simulink model "clusterDemo"  (Simulink 7.4)
settings: Solver=ode45  StartTime=0.0  StopTime=10.0  RelTol=1e-3
values from neighbouring files (symbols this model uses):
  A = 1    [clusterDemo.mat]
  B = [-1 -1 -1 -1 -1 -1 -1 -1 -1 -1 -1 -1 ... (21 elements, 1x21)]    [clusterDemo.mat]
  C = 1    [clusterDemo.mat]
  D = [0 0 0 0 0 0 0 0 0 0 0 0 ... (21 elements, 1x21)]    [clusterDemo.mat]
  N = 5    [clusterDemo.mat]    (also in firefliesDemo.mat = 10)
  var = 0    [clusterDemo.mat]    (also in firefliesDemo.mat = 3)
  x0 = 80    [clusterDemo.mat]
(part 1 of 4)
settings Model: Creator=chepeadan  LastModifiedBy=chepeadan
settings DataIOCC: SaveOutput=off  SaveState=on

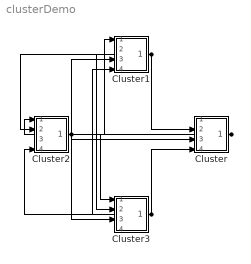
== system clusterDemo ==
  Cluster : Subsystem
  Cluster1 : Subsystem
  Cluster2 : Subsystem
  Cluster3 : Subsystem
  wires:
  Cluster/1(Out1) -> Cluster1/1(In1), Cluster2/1(In1), Cluster3/1(In1)
  Cluster1/1(Out1) -> Cluster/2(In2), Cluster2/2(In2), Cluster3/2(In2)
  Cluster2/1(Out1) -> Cluster/3(In3), Cluster1/3(In3), Cluster3/3(In3)
  Cluster3/1(Out1) -> Cluster/4(In4), Cluster1/4(In4), Cluster2/4(In4)

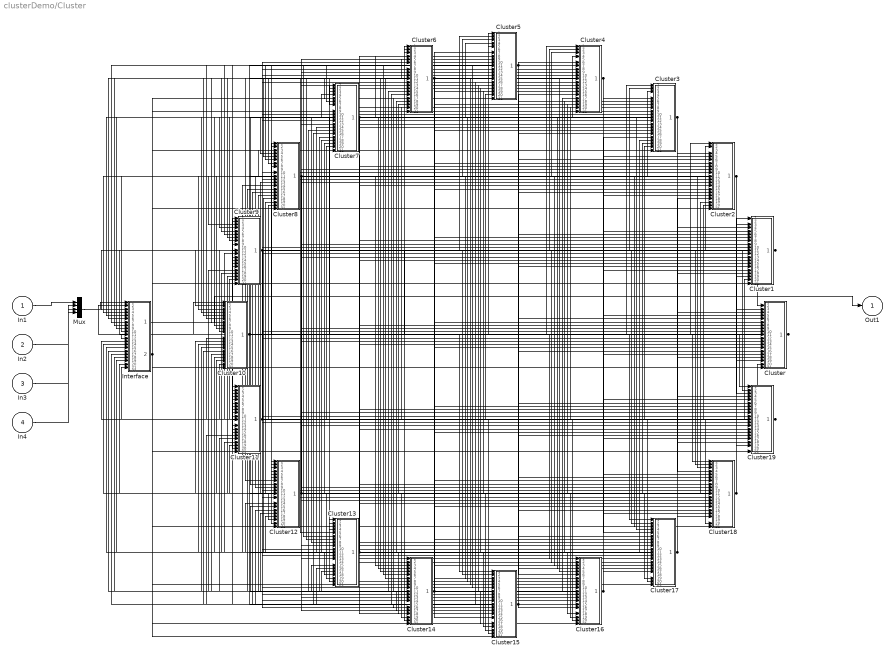
== system clusterDemo/Cluster ==
  In1 : Inport
  In2 : Inport  Port=2
  In3 : Inport  Port=3
  In4 : Inport  Port=4
  Cluster : Subsystem
  Cluster1 : Subsystem
  Cluster10 : Subsystem
  Cluster11 : Subsystem
  Cluster12 : Subsystem
  Cluster13 : Subsystem
  Cluster14 : Subsystem
  Cluster15 : Subsystem
  Cluster16 : Subsystem
  Cluster17 : Subsystem
  Cluster18 : Subsystem
  Cluster19 : Subsystem
  Cluster2 : Subsystem
  Cluster3 : Subsystem
  Cluster4 : Subsystem
  Cluster5 : Subsystem
  Cluster6 : Subsystem
  Cluster7 : Subsystem
  Cluster8 : Subsystem
  Cluster9 : Subsystem
  Interface : Subsystem
  Mux : Mux
  Out1 : Outport
  wires:
  In4/1 -> Mux/4
  In3/1 -> Mux/3
  In2/1 -> Mux/2
  Interface/1(layerOut) -> Out1/1
  Interface/2(Out1) -> Cluster19/21(In21), Cluster18/21(In21), Cluster17/21(In21), Cluster16/21(In21), Cluster15/21(In21), Cluster14/21(In21), Cluster13/21(In21), Cluster12/21(In21), Cluster11/21(In21), Cluster10/21(In21), Cluster9/21(In21), Cluster8/21(In21), Cluster7/21(In21), Cluster6/21(In21), Cluster5/21(In21), Cluster4/21(In21), Cluster3/21(In21), Cluster2/21(In21), Cluster1/21(In21), Cluster/21(In21)
  Cluster19/1(Out1) -> Interface/21(In20), Cluster18/20(In20), Cluster17/20(In20), Cluster16/20(In20), Cluster15/20(In20), Cluster14/20(In20), Cluster13/20(In20), Cluster12/20(In20), Cluster11/20(In20), Cluster10/20(In20), Cluster9/20(In20), Cluster8/20(In20), Cluster7/20(In20), Cluster6/20(In20), Cluster5/20(In20), Cluster4/20(In20), Cluster3/20(In20), Cluster2/20(In20), Cluster1/20(In20), Cluster/20(In20)
  Cluster18/1(Out1) -> Interface/20(In19), Cluster19/19(In19), Cluster17/19(In19), Cluster16/19(In19), Cluster15/19(In19), Cluster14/19(In19), Cluster13/19(In19), Cluster12/19(In19), Cluster11/19(In19), Cluster10/19(In19), Cluster9/19(In19), Cluster8/19(In19), Cluster7/19(In19), Cluster6/19(In19), Cluster5/19(In19), Cluster4/19(In19), Cluster3/19(In19), Cluster2/19(In19), Cluster1/19(In19), Cluster/19(In19)
  Cluster17/1(Out1) -> Interface/19(In18), Cluster19/18(In18), Cluster18/18(In18), Cluster16/18(In18), Cluster15/18(In18), Cluster14/18(In18), Cluster13/18(In18), Cluster12/18(In18), Cluster11/18(In18), Cluster10/18(In18), Cluster9/18(In18), Cluster8/18(In18), Cluster7/18(In18), Cluster6/18(In18), Cluster5/18(In18), Cluster4/18(In18), Cluster3/18(In18), Cluster2/18(In18), Cluster1/18(In18), Cluster/18(In18)
  Cluster16/1(Out1) -> Interface/18(In17), Cluster19/17(In17), Cluster18/17(In17), Cluster17/17(In17), Cluster15/17(In17), Cluster14/17(In17), Cluster13/17(In17), Cluster12/17(In17), Cluster11/17(In17), Cluster10/17(In17), Cluster9/17(In17), Cluster8/17(In17), Cluster7/17(In17), Cluster6/17(In17), Cluster5/17(In17), Cluster4/17(In17), Cluster3/17(In17), Cluster2/17(In17), Cluster1/17(In17), Cluster/17(In17)
  Cluster15/1(Out1) -> Interface/17(In16), Cluster19/16(In16), Cluster18/16(In16), Cluster17/16(In16), Cluster16/16(In16), Cluster14/16(In16), Cluster13/16(In16), Cluster12/16(In16), Cluster11/16(In16), Cluster10/16(In16), Cluster9/16(In16), Cluster8/16(In16), Cluster7/16(In16), Cluster6/16(In16), Cluster5/16(In16), Cluster4/16(In16), Cluster3/16(In16), Cluster2/16(In16), Cluster1/16(In16), Cluster/16(In16)
  Cluster14/1(Out1) -> Interface/16(In15), Cluster19/15(In15), Cluster18/15(In15), Cluster17/15(In15), Cluster16/15(In15), Cluster15/15(In15), Cluster13/15(In15), Cluster12/15(In15), Cluster11/15(In15), Cluster10/15(In15), Cluster9/15(In15), Cluster8/15(In15), Cluster7/15(In15), Cluster6/15(In15), Cluster5/15(In15), Cluster4/15(In15), Cluster3/15(In15), Cluster2/15(In15), Cluster1/15(In15), Cluster/15(In15)
  Cluster13/1(Out1) -> Interface/15(In14), Cluster19/14(In14), Cluster18/14(In14), Cluster17/14(In14), Cluster16/14(In14), Cluster15/14(In14), Cluster14/14(In14), Cluster12/14(In14), Cluster11/14(In14), Cluster10/14(In14), Cluster9/14(In14), Cluster8/14(In14), Cluster7/14(In14), Cluster6/14(In14), Cluster5/14(In14), Cluster4/14(In14), Cluster3/14(In14), Cluster2/14(In14), Cluster1/14(In14), Cluster/14(In14)
  Cluster12/1(Out1) -> Interface/14(In13), Cluster19/13(In13), Cluster18/13(In13), Cluster17/13(In13), Cluster16/13(In13), Cluster15/13(In13), Cluster14/13(In13), Cluster13/13(In13), Cluster11/13(In13), Cluster10/13(In13), Cluster9/13(In13), Cluster8/13(In13), Cluster7/13(In13), Cluster6/13(In13), Cluster5/13(In13), Cluster4/13(In13), Cluster3/13(In13), Cluster2/13(In13), Cluster1/13(In13), Cluster/13(In13)
  Cluster11/1(Out1) -> Interface/13(In12), Cluster19/12(In12), Cluster18/12(In12), Cluster17/12(In12), Cluster16/12(In12), Cluster15/12(In12), Cluster14/12(In12), Cluster13/12(In12), Cluster12/12(In12), Cluster10/12(In12), Cluster9/12(In12), Cluster8/12(In12), Cluster7/12(In12), Cluster6/12(In12), Cluster5/12(In12), Cluster4/12(In12), Cluster3/12(In12), Cluster2/12(In12), Cluster1/12(In12), Cluster/12(In12)
  Cluster10/1(Out1) -> Interface/12(In11), Cluster19/11(In11), Cluster18/11(In11), Cluster17/11(In11), Cluster16/11(In11), Cluster15/11(In11), Cluster14/11(In11), Cluster13/11(In11), Cluster12/11(In11), Cluster11/11(In11), Cluster9/11(In11), Cluster8/11(In11), Cluster7/11(In11), Cluster6/11(In11), Cluster5/11(In11), Cluster4/11(In11), Cluster3/11(In11), Cluster2/11(In11), Cluster1/11(In11), Cluster/11(In11)
  Cluster9/1(Out1) -> Interface/11(In10), Cluster19/10(In10), Cluster18/10(In10), Cluster17/10(In10), Cluster16/10(In10), Cluster15/10(In10), Cluster14/10(In10), Cluster13/10(In10), Cluster12/10(In10), Cluster11/10(In10), Cluster10/10(In10), Cluster8/10(In10), Cluster7/10(In10), Cluster6/10(In10), Cluster5/10(In10), Cluster4/10(In10), Cluster3/10(In10), Cluster2/10(In10), Cluster1/10(In10), Cluster/10(In10)
  Cluster8/1(Out1) -> Interface/10(In9), Cluster19/9(In9), Cluster18/9(In9), Cluster17/9(In9), Cluster16/9(In9), Cluster15/9(In9), Cluster14/9(In9), Cluster13/9(In9), Cluster12/9(In9), Cluster11/9(In9), Cluster10/9(In9), Cluster9/9(In9), Cluster7/9(In9), Cluster6/9(In9), Cluster5/9(In9), Cluster4/9(In9), Cluster3/9(In9), Cluster2/9(In9), Cluster1/9(In9), Cluster/9(In9)
  Cluster7/1(Out1) -> Interface/9(In8), Cluster19/8(In8), Cluster18/8(In8), Cluster17/8(In8), Cluster16/8(In8), Cluster15/8(In8), Cluster14/8(In8), Cluster13/8(In8), Cluster12/8(In8), Cluster11/8(In8), Cluster10/8(In8), Cluster9/8(In8), Cluster8/8(In8), Cluster6/8(In8), Cluster5/8(In8), Cluster4/8(In8), Cluster3/8(In8), Cluster2/8(In8), Cluster1/8(In8), Cluster/8(In8)
  Cluster6/1(Out1) -> Interface/8(In7), Cluster19/7(In7), Cluster18/7(In7), Cluster17/7(In7), Cluster16/7(In7), Cluster15/7(In7), Cluster14/7(In7), Cluster13/7(In7), Cluster12/7(In7), Cluster11/7(In7), Cluster10/7(In7), Cluster9/7(In7), Cluster8/7(In7), Cluster7/7(In7), Cluster5/7(In7), Cluster4/7(In7), Cluster3/7(In7), Cluster2/7(In7), Cluster1/7(In7), Cluster/7(In7)
  Cluster5/1(Out1) -> Interface/7(In6), Cluster19/6(In6), Cluster18/6(In6), Cluster17/6(In6), Cluster16/6(In6), Cluster15/6(In6), Cluster14/6(In6), Cluster13/6(In6), Cluster12/6(In6), Cluster11/6(In6), Cluster10/6(In6), Cluster9/6(In6), Cluster8/6(In6), Cluster7/6(In6), Cluster6/6(In6), Cluster4/6(In6), Cluster3/6(In6), Cluster2/6(In6), Cluster1/6(In6), Cluster/6(In6)
  Cluster4/1(Out1) -> Interface/6(In5), Cluster19/5(In5), Cluster18/5(In5), Cluster17/5(In5), Cluster16/5(In5), Cluster15/5(In5), Cluster14/5(In5), Cluster13/5(In5), Cluster12/5(In5), Cluster11/5(In5), Cluster10/5(In5), Cluster9/5(In5), Cluster8/5(In5), Cluster7/5(In5), Cluster6/5(In5), Cluster5/5(In5), Cluster3/5(In5), Cluster2/5(In5), Cluster1/5(In5), Cluster/5(In5)
  Cluster3/1(Out1) -> Interface/5(In4), Cluster19/4(In4), Cluster18/4(In4), Cluster17/4(In4), Cluster16/4(In4), Cluster15/4(In4), Cluster14/4(In4), Cluster13/4(In4), Cluster12/4(In4), Cluster11/4(In4), Cluster10/4(In4), Cluster9/4(In4), Cluster8/4(In4), Cluster7/4(In4), Cluster6/4(In4), Cluster5/4(In4), Cluster4/4(In4), Cluster2/4(In4), Cluster1/4(In4), Cluster/4(In4)
  Cluster2/1(Out1) -> Interface/4(In3), Cluster19/3(In3), Cluster18/3(In3), Cluster17/3(In3), Cluster16/3(In3), Cluster15/3(In3), Cluster14/3(In3), Cluster13/3(In3), Cluster12/3(In3), Cluster11/3(In3), Cluster10/3(In3), Cluster9/3(In3), Cluster8/3(In3), Cluster7/3(In3), Cluster6/3(In3), Cluster5/3(In3), Cluster4/3(In3), Cluster3/3(In3), Cluster1/3(In3), Cluster/3(In3)
  Cluster1/1(Out1) -> Interface/3(In2), Cluster19/2(In2), Cluster18/2(In2), Cluster17/2(In2), Cluster16/2(In2), Cluster15/2(In2), Cluster14/2(In2), Cluster13/2(In2), Cluster12/2(In2), Cluster11/2(In2), Cluster10/2(In2), Cluster9/2(In2), Cluster8/2(In2), Cluster7/2(In2), Cluster6/2(In2), Cluster5/2(In2), Cluster4/2(In2), Cluster3/2(In2), Cluster2/2(In2), Cluster/2(In2)
  Cluster/1(Out1) -> Interface/2(In1), Cluster19/1(In1), Cluster18/1(In1), Cluster17/1(In1), Cluster16/1(In1), Cluster15/1(In1), Cluster14/1(In1), Cluster13/1(In1), Cluster12/1(In1), Cluster11/1(In1), Cluster10/1(In1), Cluster9/1(In1), Cluster8/1(In1), Cluster7/1(In1), Cluster6/1(In1), Cluster5/1(In1), Cluster4/1(In1), Cluster3/1(In1), Cluster2/1(In1), Cluster1/1(In1)
  In1/1 -> Mux/1
  Mux/1 -> Interface/1(layerIn)

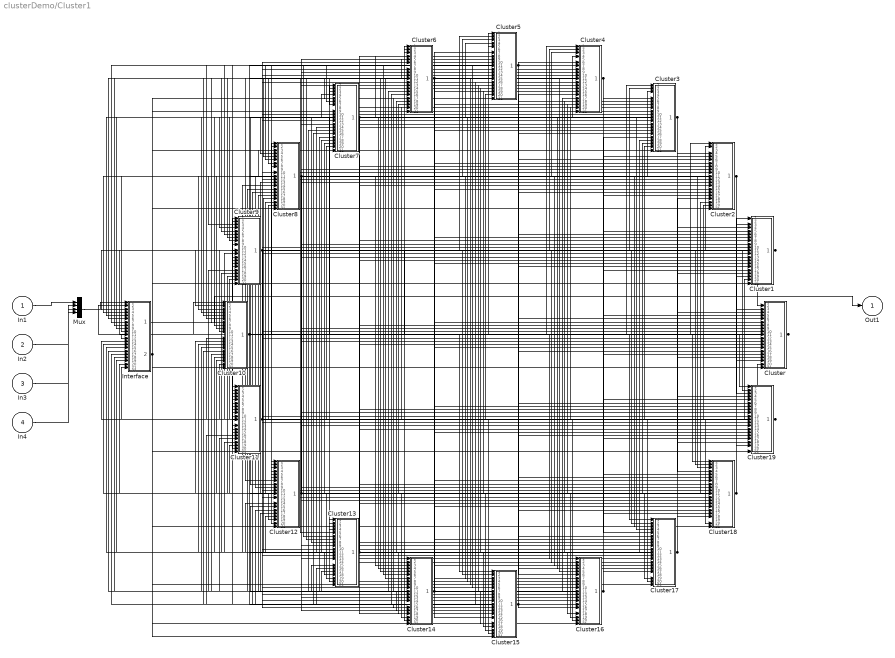
== system clusterDemo/Cluster1 ==
  In1 : Inport
  In2 : Inport  Port=2
  In3 : Inport  Port=3
  In4 : Inport  Port=4
  Cluster : Subsystem
  Cluster1 : Subsystem
  Cluster10 : Subsystem
  Cluster11 : Subsystem
  Cluster12 : Subsystem
  Cluster13 : Subsystem
  Cluster14 : Subsystem
  Cluster15 : Subsystem
  Cluster16 : Subsystem
  Cluster17 : Subsystem
  Cluster18 : Subsystem
  Cluster19 : Subsystem
  Cluster2 : Subsystem
  Cluster3 : Subsystem
  Cluster4 : Subsystem
  Cluster5 : Subsystem
  Cluster6 : Subsystem
  Cluster7 : Subsystem
  Cluster8 : Subsystem
  Cluster9 : Subsystem
  Interface : Subsystem
  Mux : Mux
  Out1 : Outport
  wires:
  In4/1 -> Mux/4
  In3/1 -> Mux/3
  In2/1 -> Mux/2
  Interface/1(layerOut) -> Out1/1
  Interface/2(Out1) -> Cluster19/21(In21), Cluster18/21(In21), Cluster17/21(In21), Cluster16/21(In21), Cluster15/21(In21), Cluster14/21(In21), Cluster13/21(In21), Cluster12/21(In21), Cluster11/21(In21), Cluster10/21(In21), Cluster9/21(In21), Cluster8/21(In21), Cluster7/21(In21), Cluster6/21(In21), Cluster5/21(In21), Cluster4/21(In21), Cluster3/21(In21), Cluster2/21(In21), Cluster1/21(In21), Cluster/21(In21)
  Cluster19/1(Out1) -> Interface/21(In20), Cluster18/20(In20), Cluster17/20(In20), Cluster16/20(In20), Cluster15/20(In20), Cluster14/20(In20), Cluster13/20(In20), Cluster12/20(In20), Cluster11/20(In20), Cluster10/20(In20), Cluster9/20(In20), Cluster8/20(In20), Cluster7/20(In20), Cluster6/20(In20), Cluster5/20(In20), Cluster4/20(In20), Cluster3/20(In20), Cluster2/20(In20), Cluster1/20(In20), Cluster/20(In20)
  Cluster18/1(Out1) -> Interface/20(In19), Cluster19/19(In19), Cluster17/19(In19), Cluster16/19(In19), Cluster15/19(In19), Cluster14/19(In19), Cluster13/19(In19), Cluster12/19(In19), Cluster11/19(In19), Cluster10/19(In19), Cluster9/19(In19), Cluster8/19(In19), Cluster7/19(In19), Cluster6/19(In19), Cluster5/19(In19), Cluster4/19(In19), Cluster3/19(In19), Cluster2/19(In19), Cluster1/19(In19), Cluster/19(In19)
  Cluster17/1(Out1) -> Interface/19(In18), Cluster19/18(In18), Cluster18/18(In18), Cluster16/18(In18), Cluster15/18(In18), Cluster14/18(In18), Cluster13/18(In18), Cluster12/18(In18), Cluster11/18(In18), Cluster10/18(In18), Cluster9/18(In18), Cluster8/18(In18), Cluster7/18(In18), Cluster6/18(In18), Cluster5/18(In18), Cluster4/18(In18), Cluster3/18(In18), Cluster2/18(In18), Cluster1/18(In18), Cluster/18(In18)
  Cluster16/1(Out1) -> Interface/18(In17), Cluster19/17(In17), Cluster18/17(In17), Cluster17/17(In17), Cluster15/17(In17), Cluster14/17(In17), Cluster13/17(In17), Cluster12/17(In17), Cluster11/17(In17), Cluster10/17(In17), Cluster9/17(In17), Cluster8/17(In17), Cluster7/17(In17), Cluster6/17(In17), Cluster5/17(In17), Cluster4/17(In17), Cluster3/17(In17), Cluster2/17(In17), Cluster1/17(In17), Cluster/17(In17)
  Cluster15/1(Out1) -> Interface/17(In16), Cluster19/16(In16), Cluster18/16(In16), Cluster17/16(In16), Cluster16/16(In16), Cluster14/16(In16), Cluster13/16(In16), Cluster12/16(In16), Cluster11/16(In16), Cluster10/16(In16), Cluster9/16(In16), Cluster8/16(In16), Cluster7/16(In16), Cluster6/16(In16), Cluster5/16(In16), Cluster4/16(In16), Cluster3/16(In16), Cluster2/16(In16), Cluster1/16(In16), Cluster/16(In16)
  Cluster14/1(Out1) -> Interface/16(In15), Cluster19/15(In15), Cluster18/15(In15), Cluster17/15(In15), Cluster16/15(In15), Cluster15/15(In15), Cluster13/15(In15), Cluster12/15(In15), Cluster11/15(In15), Cluster10/15(In15), Cluster9/15(In15), Cluster8/15(In15), Cluster7/15(In15), Cluster6/15(In15), Cluster5/15(In15), Cluster4/15(In15), Cluster3/15(In15), Cluster2/15(In15), Cluster1/15(In15), Cluster/15(In15)
  Cluster13/1(Out1) -> Interface/15(In14), Cluster19/14(In14), Cluster18/14(In14), Cluster17/14(In14), Cluster16/14(In14), Cluster15/14(In14), Cluster14/14(In14), Cluster12/14(In14), Cluster11/14(In14), Cluster10/14(In14), Cluster9/14(In14), Cluster8/14(In14), Cluster7/14(In14), Cluster6/14(In14), Cluster5/14(In14), Cluster4/14(In14), Cluster3/14(In14), Cluster2/14(In14), Cluster1/14(In14), Cluster/14(In14)
  Cluster12/1(Out1) -> Interface/14(In13), Cluster19/13(In13), Cluster18/13(In13), Cluster17/13(In13), Cluster16/13(In13), Cluster15/13(In13), Cluster14/13(In13), Cluster13/13(In13), Cluster11/13(In13), Cluster10/13(In13), Cluster9/13(In13), Cluster8/13(In13), Cluster7/13(In13), Cluster6/13(In13), Cluster5/13(In13), Cluster4/13(In13), Cluster3/13(In13), Cluster2/13(In13), Cluster1/13(In13), Cluster/13(In13)
  Cluster11/1(Out1) -> Interface/13(In12), Cluster19/12(In12), Cluster18/12(In12), Cluster17/12(In12), Cluster16/12(In12), Cluster15/12(In12), Cluster14/12(In12), Cluster13/12(In12), Cluster12/12(In12), Cluster10/12(In12), Cluster9/12(In12), Cluster8/12(In12), Cluster7/12(In12), Cluster6/12(In12), Cluster5/12(In12), Cluster4/12(In12), Cluster3/12(In12), Cluster2/12(In12), Cluster1/12(In12), Cluster/12(In12)
  Cluster10/1(Out1) -> Interface/12(In11), Cluster19/11(In11), Cluster18/11(In11), Cluster17/11(In11), Cluster16/11(In11), Cluster15/11(In11), Cluster14/11(In11), Cluster13/11(In11), Cluster12/11(In11), Cluster11/11(In11), Cluster9/11(In11), Cluster8/11(In11), Cluster7/11(In11), Cluster6/11(In11), Cluster5/11(In11), Cluster4/11(In11), Cluster3/11(In11), Cluster2/11(In11), Cluster1/11(In11), Cluster/11(In11)
  Cluster9/1(Out1) -> Interface/11(In10), Cluster19/10(In10), Cluster18/10(In10), Cluster17/10(In10), Cluster16/10(In10), Cluster15/10(In10), Cluster14/10(In10), Cluster13/10(In10), Cluster12/10(In10), Cluster11/10(In10), Cluster10/10(In10), Cluster8/10(In10), Cluster7/10(In10), Cluster6/10(In10), Cluster5/10(In10), Cluster4/10(In10), Cluster3/10(In10), Cluster2/10(In10), Cluster1/10(In10), Cluster/10(In10)
  Cluster8/1(Out1) -> Interface/10(In9), Cluster19/9(In9), Cluster18/9(In9), Cluster17/9(In9), Cluster16/9(In9), Cluster15/9(In9), Cluster14/9(In9), Cluster13/9(In9), Cluster12/9(In9), Cluster11/9(In9), Cluster10/9(In9), Cluster9/9(In9), Cluster7/9(In9), Cluster6/9(In9), Cluster5/9(In9), Cluster4/9(In9), Cluster3/9(In9), Cluster2/9(In9), Cluster1/9(In9), Cluster/9(In9)
  Cluster7/1(Out1) -> Interface/9(In8), Cluster19/8(In8), Cluster18/8(In8), Cluster17/8(In8), Cluster16/8(In8), Cluster15/8(In8), Cluster14/8(In8), Cluster13/8(In8), Cluster12/8(In8), Cluster11/8(In8), Cluster10/8(In8), Cluster9/8(In8), Cluster8/8(In8), Cluster6/8(In8), Cluster5/8(In8), Cluster4/8(In8), Cluster3/8(In8), Cluster2/8(In8), Cluster1/8(In8), Cluster/8(In8)
  Cluster6/1(Out1) -> Interface/8(In7), Cluster19/7(In7), Cluster18/7(In7), Cluster17/7(In7), Cluster16/7(In7), Cluster15/7(In7), Cluster14/7(In7), Cluster13/7(In7), Cluster12/7(In7), Cluster11/7(In7), Cluster10/7(In7), Cluster9/7(In7), Cluster8/7(In7), Cluster7/7(In7), Cluster5/7(In7), Cluster4/7(In7), Cluster3/7(In7), Cluster2/7(In7), Cluster1/7(In7), Cluster/7(In7)
  Cluster5/1(Out1) -> Interface/7(In6), Cluster19/6(In6), Cluster18/6(In6), Cluster17/6(In6), Cluster16/6(In6), Cluster15/6(In6), Cluster14/6(In6), Cluster13/6(In6), Cluster12/6(In6), Cluster11/6(In6), Cluster10/6(In6), Cluster9/6(In6), Cluster8/6(In6), Cluster7/6(In6), Cluster6/6(In6), Cluster4/6(In6), Cluster3/6(In6), Cluster2/6(In6), Cluster1/6(In6), Cluster/6(In6)
  Cluster4/1(Out1) -> Interface/6(In5), Cluster19/5(In5), Cluster18/5(In5), Cluster17/5(In5), Cluster16/5(In5), Cluster15/5(In5), Cluster14/5(In5), Cluster13/5(In5), Cluster12/5(In5), Cluster11/5(In5), Cluster10/5(In5), Cluster9/5(In5), Cluster8/5(In5), Cluster7/5(In5), Cluster6/5(In5), Cluster5/5(In5), Cluster3/5(In5), Cluster2/5(In5), Cluster1/5(In5), Cluster/5(In5)
  Cluster3/1(Out1) -> Interface/5(In4), Cluster19/4(In4), Cluster18/4(In4), Cluster17/4(In4), Cluster16/4(In4), Cluster15/4(In4), Cluster14/4(In4), Cluster13/4(In4), Cluster12/4(In4), Cluster11/4(In4), Cluster10/4(In4), Cluster9/4(In4), Cluster8/4(In4), Cluster7/4(In4), Cluster6/4(In4), Cluster5/4(In4), Cluster4/4(In4), Cluster2/4(In4), Cluster1/4(In4), Cluster/4(In4)
  Cluster2/1(Out1) -> Interface/4(In3), Cluster19/3(In3), Cluster18/3(In3), Cluster17/3(In3), Cluster16/3(In3), Cluster15/3(In3), Cluster14/3(In3), Cluster13/3(In3), Cluster12/3(In3), Cluster11/3(In3), Cluster10/3(In3), Cluster9/3(In3), Cluster8/3(In3), Cluster7/3(In3), Cluster6/3(In3), Cluster5/3(In3), Cluster4/3(In3), Cluster3/3(In3), Cluster1/3(In3), Cluster/3(In3)
  Cluster1/1(Out1) -> Interface/3(In2), Cluster19/2(In2), Cluster18/2(In2), Cluster17/2(In2), Cluster16/2(In2), Cluster15/2(In2), Cluster14/2(In2), Cluster13/2(In2), Cluster12/2(In2), Cluster11/2(In2), Cluster10/2(In2), Cluster9/2(In2), Cluster8/2(In2), Cluster7/2(In2), Cluster6/2(In2), Cluster5/2(In2), Cluster4/2(In2), Cluster3/2(In2), Cluster2/2(In2), Cluster/2(In2)
  Cluster/1(Out1) -> Interface/2(In1), Cluster19/1(In1), Cluster18/1(In1), Cluster17/1(In1), Cluster16/1(In1), Cluster15/1(In1), Cluster14/1(In1), Cluster13/1(In1), Cluster12/1(In1), Cluster11/1(In1), Cluster10/1(In1), Cluster9/1(In1), Cluster8/1(In1), Cluster7/1(In1), Cluster6/1(In1), Cluster5/1(In1), Cluster4/1(In1), Cluster3/1(In1), Cluster2/1(In1), Cluster1/1(In1)
  In1/1 -> Mux/1
  Mux/1 -> Interface/1(layerIn)

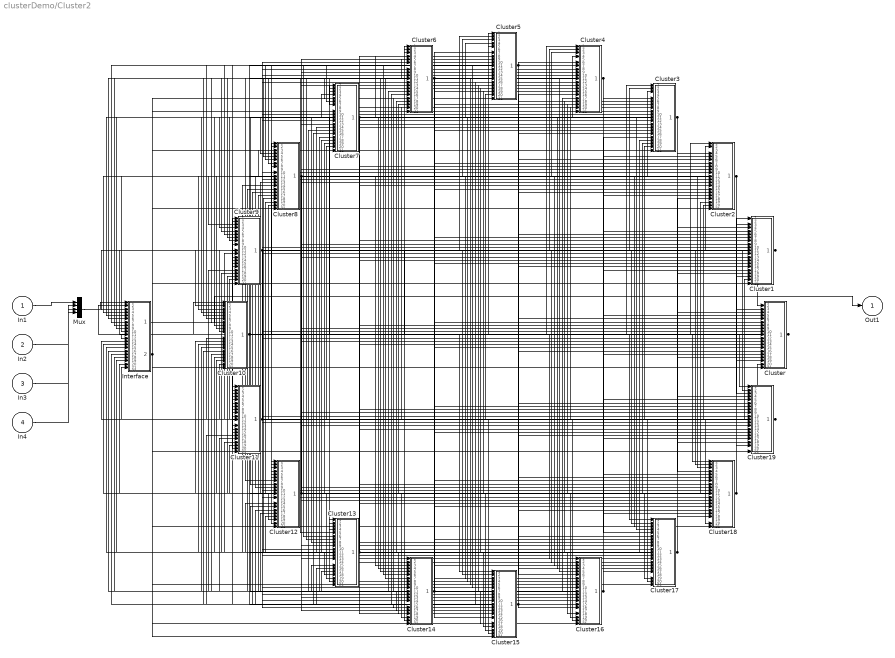
== system clusterDemo/Cluster2 ==
  In1 : Inport
  In2 : Inport  Port=2
  In3 : Inport  Port=3
  In4 : Inport  Port=4
  Cluster : Subsystem
  Cluster1 : Subsystem
  Cluster10 : Subsystem
  Cluster11 : Subsystem
  Cluster12 : Subsystem
  Cluster13 : Subsystem
  Cluster14 : Subsystem
  Cluster15 : Subsystem
  Cluster16 : Subsystem
  Cluster17 : Subsystem
  Cluster18 : Subsystem
  Cluster19 : Subsystem
  Cluster2 : Subsystem
  Cluster3 : Subsystem
  Cluster4 : Subsystem
  Cluster5 : Subsystem
  Cluster6 : Subsystem
  Cluster7 : Subsystem
  Cluster8 : Subsystem
  Cluster9 : Subsystem
  Interface : Subsystem
  Mux : Mux
  Out1 : Outport
  wires:
  In4/1 -> Mux/4
  In3/1 -> Mux/3
  In2/1 -> Mux/2
  Interface/1(layerOut) -> Out1/1
  Interface/2(Out1) -> Cluster19/21(In21), Cluster18/21(In21), Cluster17/21(In21), Cluster16/21(In21), Cluster15/21(In21), Cluster14/21(In21), Cluster13/21(In21), Cluster12/21(In21), Cluster11/21(In21), Cluster10/21(In21), Cluster9/21(In21), Cluster8/21(In21), Cluster7/21(In21), Cluster6/21(In21), Cluster5/21(In21), Cluster4/21(In21), Cluster3/21(In21), Cluster2/21(In21), Cluster1/21(In21), Cluster/21(In21)
  Cluster19/1(Out1) -> Interface/21(In20), Cluster18/20(In20), Cluster17/20(In20), Cluster16/20(In20), Cluster15/20(In20), Cluster14/20(In20), Cluster13/20(In20), Cluster12/20(In20), Cluster11/20(In20), Cluster10/20(In20), Cluster9/20(In20), Cluster8/20(In20), Cluster7/20(In20), Cluster6/20(In20), Cluster5/20(In20), Cluster4/20(In20), Cluster3/20(In20), Cluster2/20(In20), Cluster1/20(In20), Cluster/20(In20)
  Cluster18/1(Out1) -> Interface/20(In19), Cluster19/19(In19), Cluster17/19(In19), Cluster16/19(In19), Cluster15/19(In19), Cluster14/19(In19), Cluster13/19(In19), Cluster12/19(In19), Cluster11/19(In19), Cluster10/19(In19), Cluster9/19(In19), Cluster8/19(In19), Cluster7/19(In19), Cluster6/19(In19), Cluster5/19(In19), Cluster4/19(In19), Cluster3/19(In19), Cluster2/19(In19), Cluster1/19(In19), Cluster/19(In19)
  Cluster17/1(Out1) -> Interface/19(In18), Cluster19/18(In18), Cluster18/18(In18), Cluster16/18(In18), Cluster15/18(In18), Cluster14/18(In18), Cluster13/18(In18), Cluster12/18(In18), Cluster11/18(In18), Cluster10/18(In18), Cluster9/18(In18), Cluster8/18(In18), Cluster7/18(In18), Cluster6/18(In18), Cluster5/18(In18), Cluster4/18(In18), Cluster3/18(In18), Cluster2/18(In18), Cluster1/18(In18), Cluster/18(In18)
  Cluster16/1(Out1) -> Interface/18(In17), Cluster19/17(In17), Cluster18/17(In17), Cluster17/17(In17), Cluster15/17(In17), Cluster14/17(In17), Cluster13/17(In17), Cluster12/17(In17), Cluster11/17(In17), Cluster10/17(In17), Cluster9/17(In17), Cluster8/17(In17), Cluster7/17(In17), Cluster6/17(In17), Cluster5/17(In17), Cluster4/17(In17), Cluster3/17(In17), Cluster2/17(In17), Cluster1/17(In17), Cluster/17(In17)
  Cluster15/1(Out1) -> Interface/17(In16), Cluster19/16(In16), Cluster18/16(In16), Cluster17/16(In16), Cluster16/16(In16), Cluster14/16(In16), Cluster13/16(In16), Cluster12/16(In16), Cluster11/16(In16), Cluster10/16(In16), Cluster9/16(In16), Cluster8/16(In16), Cluster7/16(In16), Cluster6/16(In16), Cluster5/16(In16), Cluster4/16(In16), Cluster3/16(In16), Cluster2/16(In16), Cluster1/16(In16), Cluster/16(In16)
  Cluster14/1(Out1) -> Interface/16(In15), Cluster19/15(In15), Cluster18/15(In15), Cluster17/15(In15), Cluster16/15(In15), Cluster15/15(In15), Cluster13/15(In15), Cluster12/15(In15), Cluster11/15(In15), Cluster10/15(In15), Cluster9/15(In15), Cluster8/15(In15), Cluster7/15(In15), Cluster6/15(In15), Cluster5/15(In15), Cluster4/15(In15), Cluster3/15(In15), Cluster2/15(In15), Cluster1/15(In15), Cluster/15(In15)
  Cluster13/1(Out1) -> Interface/15(In14), Cluster19/14(In14), Cluster18/14(In14), Cluster17/14(In14), Cluster16/14(In14), Cluster15/14(In14), Cluster14/14(In14), Cluster12/14(In14), Cluster11/14(In14), Cluster10/14(In14), Cluster9/14(In14), Cluster8/14(In14), Cluster7/14(In14), Cluster6/14(In14), Cluster5/14(In14), Cluster4/14(In14), Cluster3/14(In14), Cluster2/14(In14), Cluster1/14(In14), Cluster/14(In14)
  Cluster12/1(Out1) -> Interface/14(In13), Cluster19/13(In13), Cluster18/13(In13), Cluster17/13(In13), Cluster16/13(In13), Cluster15/13(In13), Cluster14/13(In13), Cluster13/13(In13), Cluster11/13(In13), Cluster10/13(In13), Cluster9/13(In13), Cluster8/13(In13), Cluster7/13(In13), Cluster6/13(In13), Cluster5/13(In13), Cluster4/13(In13), Cluster3/13(In13), Cluster2/13(In13), Cluster1/13(In13), Cluster/13(In13)
  Cluster11/1(Out1) -> Interface/13(In12), Cluster19/12(In12), Cluster18/12(In12), Cluster17/12(In12), Cluster16/12(In12), Cluster15/12(In12), Cluster14/12(In12), Cluster13/12(In12), Cluster12/12(In12), Cluster10/12(In12), Cluster9/12(In12), Cluster8/12(In12), Cluster7/12(In12), Cluster6/12(In12), Cluster5/12(In12), Cluster4/12(In12), Cluster3/12(In12), Cluster2/12(In12), Cluster1/12(In12), Cluster/12(In12)
  Cluster10/1(Out1) -> Interface/12(In11), Cluster19/11(In11), Cluster18/11(In11), Cluster17/11(In11), Cluster16/11(In11), Cluster15/11(In11), Cluster14/11(In11), Cluster13/11(In11), Cluster12/11(In11), Cluster11/11(In11), Cluster9/11(In11), Cluster8/11(In11), Cluster7/11(In11), Cluster6/11(In11), Cluster5/11(In11), Cluster4/11(In11), Cluster3/11(In11), Cluster2/11(In11), Cluster1/11(In11), Cluster/11(In11)
  Cluster9/1(Out1) -> Interface/11(In10), Cluster19/10(In10), Cluster18/10(In10), Cluster17/10(In10), Cluster16/10(In10), Cluster15/10(In10), Cluster14/10(In10), Cluster13/10(In10), Cluster12/10(In10), Cluster11/10(In10), Cluster10/10(In10), Cluster8/10(In10), Cluster7/10(In10), Cluster6/10(In10), Cluster5/10(In10), Cluster4/10(In10), Cluster3/10(In10), Cluster2/10(In10), Cluster1/10(In10), Cluster/10(In10)
  Cluster8/1(Out1) -> Interface/10(In9), Cluster19/9(In9), Cluster18/9(In9), Cluster17/9(In9), Cluster16/9(In9), Cluster15/9(In9), Cluster14/9(In9), Cluster13/9(In9), Cluster12/9(In9), Cluster11/9(In9), Cluster10/9(In9), Cluster9/9(In9), Cluster7/9(In9), Cluster6/9(In9), Cluster5/9(In9), Cluster4/9(In9), Cluster3/9(In9), Cluster2/9(In9), Cluster1/9(In9), Cluster/9(In9)
  Cluster7/1(Out1) -> Interface/9(In8), Cluster19/8(In8), Cluster18/8(In8), Cluster17/8(In8), Cluster16/8(In8), Cluster15/8(In8), Cluster14/8(In8), Cluster13/8(In8), Cluster12/8(In8), Cluster11/8(In8), Cluster10/8(In8), Cluster9/8(In8), Cluster8/8(In8), Cluster6/8(In8), Cluster5/8(In8), Cluster4/8(In8), Cluster3/8(In8), Cluster2/8(In8), Cluster1/8(In8), Cluster/8(In8)
  Cluster6/1(Out1) -> Interface/8(In7), Cluster19/7(In7), Cluster18/7(In7), Cluster17/7(In7), Cluster16/7(In7), Cluster15/7(In7), Cluster14/7(In7), Cluster13/7(In7), Cluster12/7(In7), Cluster11/7(In7), Cluster10/7(In7), Cluster9/7(In7), Cluster8/7(In7), Cluster7/7(In7), Cluster5/7(In7), Cluster4/7(In7), Cluster3/7(In7), Cluster2/7(In7), Cluster1/7(In7), Cluster/7(In7)
  Cluster5/1(Out1) -> Interface/7(In6), Cluster19/6(In6), Cluster18/6(In6), Cluster17/6(In6), Cluster16/6(In6), Cluster15/6(In6), Cluster14/6(In6), Cluster13/6(In6), Cluster12/6(In6), Cluster11/6(In6), Cluster10/6(In6), Cluster9/6(In6), Cluster8/6(In6), Cluster7/6(In6), Cluster6/6(In6), Cluster4/6(In6), Cluster3/6(In6), Cluster2/6(In6), Cluster1/6(In6), Cluster/6(In6)
  Cluster4/1(Out1) -> Interface/6(In5), Cluster19/5(In5), Cluster18/5(In5), Cluster17/5(In5), Cluster16/5(In5), Cluster15/5(In5), Cluster14/5(In5), Cluster13/5(In5), Cluster12/5(In5), Cluster11/5(In5), Cluster10/5(In5), Cluster9/5(In5), Cluster8/5(In5), Cluster7/5(In5), Cluster6/5(In5), Cluster5/5(In5), Cluster3/5(In5), Cluster2/5(In5), Cluster1/5(In5), Cluster/5(In5)
  Cluster3/1(Out1) -> Interface/5(In4), Cluster19/4(In4), Cluster18/4(In4), Cluster17/4(In4), Cluster16/4(In4), Cluster15/4(In4), Cluster14/4(In4), Cluster13/4(In4), Cluster12/4(In4), Cluster11/4(In4), Cluster10/4(In4), Cluster9/4(In4), Cluster8/4(In4), Cluster7/4(In4), Cluster6/4(In4), Cluster5/4(In4), Cluster4/4(In4), Cluster2/4(In4), Cluster1/4(In4), Cluster/4(In4)
  Cluster2/1(Out1) -> Interface/4(In3), Cluster19/3(In3), Cluster18/3(In3), Cluster17/3(In3), Cluster16/3(In3), Cluster15/3(In3), Cluster14/3(In3), Cluster13/3(In3), Cluster12/3(In3), Cluster11/3(In3), Cluster10/3(In3), Cluster9/3(In3), Cluster8/3(In3), Cluster7/3(In3), Cluster6/3(In3), Cluster5/3(In3), Cluster4/3(In3), Cluster3/3(In3), Cluster1/3(In3), Cluster/3(In3)
  Cluster1/1(Out1) -> Interface/3(In2), Cluster19/2(In2), Cluster18/2(In2), Cluster17/2(In2), Cluster16/2(In2), Cluster15/2(In2), Cluster14/2(In2), Cluster13/2(In2), Cluster12/2(In2), Cluster11/2(In2), Cluster10/2(In2), Cluster9/2(In2), Cluster8/2(In2), Cluster7/2(In2), Cluster6/2(In2), Cluster5/2(In2), Cluster4/2(In2), Cluster3/2(In2), Cluster2/2(In2), Cluster/2(In2)
  Cluster/1(Out1) -> Interface/2(In1), Cluster19/1(In1), Cluster18/1(In1), Cluster17/1(In1), Cluster16/1(In1), Cluster15/1(In1), Cluster14/1(In1), Cluster13/1(In1), Cluster12/1(In1), Cluster11/1(In1), Cluster10/1(In1), Cluster9/1(In1), Cluster8/1(In1), Cluster7/1(In1), Cluster6/1(In1), Cluster5/1(In1), Cluster4/1(In1), Cluster3/1(In1), Cluster2/1(In1), Cluster1/1(In1)
  In1/1 -> Mux/1
  Mux/1 -> Interface/1(layerIn)

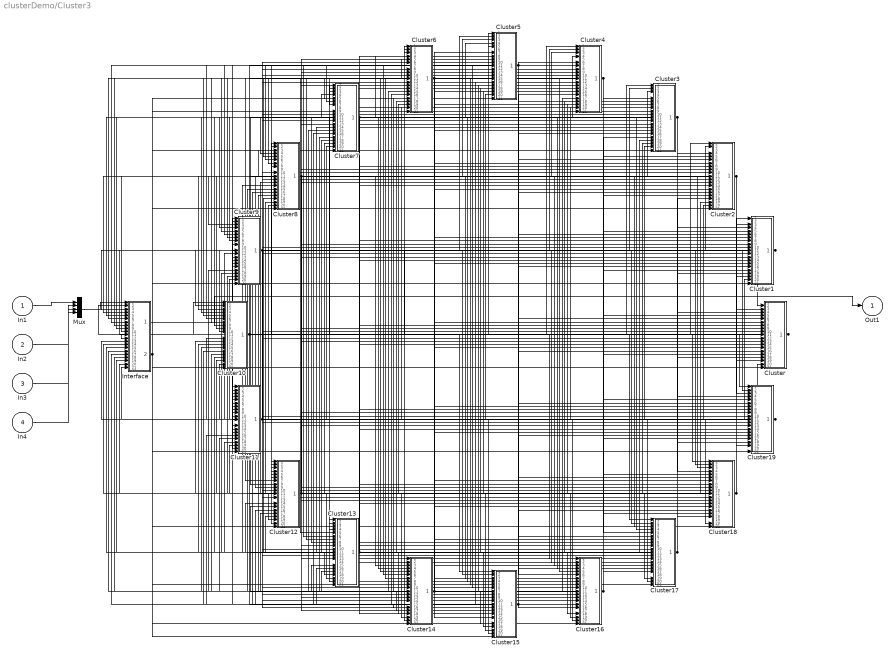
== system clusterDemo/Cluster3 ==
  In1 : Inport
  In2 : Inport  Port=2
  In3 : Inport  Port=3
  In4 : Inport  Port=4
  Cluster : Subsystem
  Cluster1 : Subsystem
  Cluster10 : Subsystem
  Cluster11 : Subsystem
  Cluster12 : Subsystem
  Cluster13 : Subsystem
  Cluster14 : Subsystem
  Cluster15 : Subsystem
  Cluster16 : Subsystem
  Cluster17 : Subsystem
  Cluster18 : Subsystem
  Cluster19 : Subsystem
  Cluster2 : Subsystem
  Cluster3 : Subsystem
  Cluster4 : Subsystem
  Cluster5 : Subsystem
  Cluster6 : Subsystem
  Cluster7 : Subsystem
  Cluster8 : Subsystem
  Cluster9 : Subsystem
  Interface : Subsystem
  Mux : Mux
  Out1 : Outport
  wires:
  In4/1 -> Mux/4
  In3/1 -> Mux/3
  In2/1 -> Mux/2
  Interface/1(layerOut) -> Out1/1
  Interface/2(Out1) -> Cluster19/21(In21), Cluster18/21(In21), Cluster17/21(In21), Cluster16/21(In21), Cluster15/21(In21), Cluster14/21(In21), Cluster13/21(In21), Cluster12/21(In21), Cluster11/21(In21), Cluster10/21(In21), Cluster9/21(In21), Cluster8/21(In21), Cluster7/21(In21), Cluster6/21(In21), Cluster5/21(In21), Cluster4/21(In21), Cluster3/21(In21), Cluster2/21(In21), Cluster1/21(In21), Cluster/21(In21)
  Cluster19/1(Out1) -> Interface/21(In20), Cluster18/20(In20), Cluster17/20(In20), Cluster16/20(In20), Cluster15/20(In20), Cluster14/20(In20), Cluster13/20(In20), Cluster12/20(In20), Cluster11/20(In20), Cluster10/20(In20), Cluster9/20(In20), Cluster8/20(In20), Cluster7/20(In20), Cluster6/20(In20), Cluster5/20(In20), Cluster4/20(In20), Cluster3/20(In20), Cluster2/20(In20), Cluster1/20(In20), Cluster/20(In20)
  Cluster18/1(Out1) -> Interface/20(In19), Cluster19/19(In19), Cluster17/19(In19), Cluster16/19(In19), Cluster15/19(In19), Cluster14/19(In19), Cluster13/19(In19), Cluster12/19(In19), Cluster11/19(In19), Cluster10/19(In19), Cluster9/19(In19), Cluster8/19(In19), Cluster7/19(In19), Cluster6/19(In19), Cluster5/19(In19), Cluster4/19(In19), Cluster3/19(In19), Cluster2/19(In19), Cluster1/19(In19), Cluster/19(In19)
  Cluster17/1(Out1) -> Interface/19(In18), Cluster19/18(In18), Cluster18/18(In18), Cluster16/18(In18), Cluster15/18(In18), Cluster14/18(In18), Cluster13/18(In18), Cluster12/18(In18), Cluster11/18(In18), Cluster10/18(In18), Cluster9/18(In18), Cluster8/18(In18), Cluster7/18(In18), Cluster6/18(In18), Cluster5/18(In18), Cluster4/18(In18), Cluster3/18(In18), Cluster2/18(In18), Cluster1/18(In18), Cluster/18(In18)
  Cluster16/1(Out1) -> Interface/18(In17), Cluster19/17(In17), Cluster18/17(In17), Cluster17/17(In17), Cluster15/17(In17), Cluster14/17(In17), Cluster13/17(In17), Cluster12/17(In17), Cluster11/17(In17), Cluster10/17(In17), Cluster9/17(In17), Cluster8/17(In17), Cluster7/17(In17), Cluster6/17(In17), Cluster5/17(In17), Cluster4/17(In17), Cluster3/17(In17), Cluster2/17(In17), Cluster1/17(In17), Cluster/17(In17)
  Cluster15/1(Out1) -> Interface/17(In16), Cluster19/16(In16), Cluster18/16(In16), Cluster17/16(In16), Cluster16/16(In16), Cluster14/16(In16), Cluster13/16(In16), Cluster12/16(In16), Cluster11/16(In16), Cluster10/16(In16), Cluster9/16(In16), Cluster8/16(In16), Cluster7/16(In16), Cluster6/16(In16), Cluster5/16(In16), Cluster4/16(In16), Cluster3/16(In16), Cluster2/16(In16), Cluster1/16(In16), Cluster/16(In16)
  Cluster14/1(Out1) -> Interface/16(In15), Cluster19/15(In15), Cluster18/15(In15), Cluster17/15(In15), Cluster16/15(In15), Cluster15/15(In15), Cluster13/15(In15), Cluster12/15(In15), Cluster11/15(In15), Cluster10/15(In15), Cluster9/15(In15), Cluster8/15(In15), Cluster7/15(In15), Cluster6/15(In15), Cluster5/15(In15), Cluster4/15(In15), Cluster3/15(In15), Cluster2/15(In15), Cluster1/15(In15), Cluster/15(In15)
  Cluster13/1(Out1) -> Interface/15(In14), Cluster19/14(In14), Cluster18/14(In14), Cluster17/14(In14), Cluster16/14(In14), Cluster15/14(In14), Cluster14/14(In14), Cluster12/14(In14), Cluster11/14(In14), Cluster10/14(In14), Cluster9/14(In14), Cluster8/14(In14), Cluster7/14(In14), Cluster6/14(In14), Cluster5/14(In14), Cluster4/14(In14), Cluster3/14(In14), Cluster2/14(In14), Cluster1/14(In14), Cluster/14(In14)
  Cluster12/1(Out1) -> Interface/14(In13), Cluster19/13(In13), Cluster18/13(In13), Cluster17/13(In13), Cluster16/13(In13), Cluster15/13(In13), Cluster14/13(In13), Cluster13/13(In13), Cluster11/13(In13), Cluster10/13(In13), Cluster9/13(In13), Cluster8/13(In13), Cluster7/13(In13), Cluster6/13(In13), Cluster5/13(In13), Cluster4/13(In13), Cluster3/13(In13), Cluster2/13(In13), Cluster1/13(In13), Cluster/13(In13)
  Cluster11/1(Out1) -> Interface/13(In12), Cluster19/12(In12), Cluster18/12(In12), Cluster17/12(In12), Cluster16/12(In12), Cluster15/12(In12), Cluster14/12(In12), Cluster13/12(In12), Cluster12/12(In12), Cluster10/12(In12), Cluster9/12(In12), Cluster8/12(In12), Cluster7/12(In12), Cluster6/12(In12), Cluster5/12(In12), Cluster4/12(In12), Cluster3/12(In12), Cluster2/12(In12), Cluster1/12(In12), Cluster/12(In12)
  Cluster10/1(Out1) -> Interface/12(In11), Cluster19/11(In11), Cluster18/11(In11), Cluster17/11(In11), Cluster16/11(In11), Cluster15/11(In11), Cluster14/11(In11), Cluster13/11(In11), Cluster12/11(In11), Cluster11/11(In11), Cluster9/11(In11), Cluster8/11(In11), Cluster7/11(In11), Cluster6/11(In11), Cluster5/11(In11), Cluster4/11(In11), Cluster3/11(In11), Cluster2/11(In11), Cluster1/11(In11), Cluster/11(In11)
  Cluster9/1(Out1) -> Interface/11(In10), Cluster19/10(In10), Cluster18/10(In10), Cluster17/10(In10), Cluster16/10(In10), Cluster15/10(In10), Cluster14/10(In10), Cluster13/10(In10), Cluster12/10(In10), Cluster11/10(In10), Cluster10/10(In10), Cluster8/10(In10), Cluster7/10(In10), Cluster6/10(In10), Cluster5/10(In10), Cluster4/10(In10), Cluster3/10(In10), Cluster2/10(In10), Cluster1/10(In10), Cluster/10(In10)
  Cluster8/1(Out1) -> Interface/10(In9), Cluster19/9(In9), Cluster18/9(In9), Cluster17/9(In9), Cluster16/9(In9), Cluster15/9(In9), Cluster14/9(In9), Cluster13/9(In9), Cluster12/9(In9), Cluster11/9(In9), Cluster10/9(In9), Cluster9/9(In9), Cluster7/9(In9), Cluster6/9(In9), Cluster5/9(In9), Cluster4/9(In9), Cluster3/9(In9), Cluster2/9(In9), Cluster1/9(In9), Cluster/9(In9)
  Cluster7/1(Out1) -> Interface/9(In8), Cluster19/8(In8), Cluster18/8(In8), Cluster17/8(In8), Cluster16/8(In8), Cluster15/8(In8), Cluster14/8(In8), Cluster13/8(In8), Cluster12/8(In8), Cluster11/8(In8), Cluster10/8(In8), Cluster9/8(In8), Cluster8/8(In8), Cluster6/8(In8), Cluster5/8(In8), Cluster4/8(In8), Cluster3/8(In8), Cluster2/8(In8), Cluster1/8(In8), Cluster/8(In8)
  Cluster6/1(Out1) -> Interface/8(In7), Cluster19/7(In7), Cluster18/7(In7), Cluster17/7(In7), Cluster16/7(In7), Cluster15/7(In7), Cluster14/7(In7), Cluster13/7(In7), Cluster12/7(In7), Cluster11/7(In7), Cluster10/7(In7), Cluster9/7(In7), Cluster8/7(In7), Cluster7/7(In7), Cluster5/7(In7), Cluster4/7(In7), Cluster3/7(In7), Cluster2/7(In7), Cluster1/7(In7), Cluster/7(In7)
  Cluster5/1(Out1) -> Interface/7(In6), Cluster19/6(In6), Cluster18/6(In6), Cluster17/6(In6), Cluster16/6(In6), Cluster15/6(In6), Cluster14/6(In6), Cluster13/6(In6), Cluster12/6(In6), Cluster11/6(In6), Cluster10/6(In6), Cluster9/6(In6), Cluster8/6(In6), Cluster7/6(In6), Cluster6/6(In6), Cluster4/6(In6), Cluster3/6(In6), Cluster2/6(In6), Cluster1/6(In6), Cluster/6(In6)
  Cluster4/1(Out1) -> Interface/6(In5), Cluster19/5(In5), Cluster18/5(In5), Cluster17/5(In5), Cluster16/5(In5), Cluster15/5(In5), Cluster14/5(In5), Cluster13/5(In5), Cluster12/5(In5), Cluster11/5(In5), Cluster10/5(In5), Cluster9/5(In5), Cluster8/5(In5), Cluster7/5(In5), Cluster6/5(In5), Cluster5/5(In5), Cluster3/5(In5), Cluster2/5(In5), Cluster1/5(In5), Cluster/5(In5)
  Cluster3/1(Out1) -> Interface/5(In4), Cluster19/4(In4), Cluster18/4(In4), Cluster17/4(In4), Cluster16/4(In4), Cluster15/4(In4), Cluster14/4(In4), Cluster13/4(In4), Cluster12/4(In4), Cluster11/4(In4), Cluster10/4(In4), Cluster9/4(In4), Cluster8/4(In4), Cluster7/4(In4), Cluster6/4(In4), Cluster5/4(In4), Cluster4/4(In4), Cluster2/4(In4), Cluster1/4(In4), Cluster/4(In4)
  Cluster2/1(Out1) -> Interface/4(In3), Cluster19/3(In3), Cluster18/3(In3), Cluster17/3(In3), Cluster16/3(In3), Cluster15/3(In3), Cluster14/3(In3), Cluster13/3(In3), Cluster12/3(In3), Cluster11/3(In3), Cluster10/3(In3), Cluster9/3(In3), Cluster8/3(In3), Cluster7/3(In3), Cluster6/3(In3), Cluster5/3(In3), Cluster4/3(In3), Cluster3/3(In3), Cluster1/3(In3), Cluster/3(In3)
  Cluster1/1(Out1) -> Interface/3(In2), Cluster19/2(In2), Cluster18/2(In2), Cluster17/2(In2), Cluster16/2(In2), Cluster15/2(In2), Cluster14/2(In2), Cluster13/2(In2), Cluster12/2(In2), Cluster11/2(In2), Cluster10/2(In2), Cluster9/2(In2), Cluster8/2(In2), Cluster7/2(In2), Cluster6/2(In2), Cluster5/2(In2), Cluster4/2(In2), Cluster3/2(In2), Cluster2/2(In2), Cluster/2(In2)
  Cluster/1(Out1) -> Interface/2(In1), Cluster19/1(In1), Cluster18/1(In1), Cluster17/1(In1), Cluster16/1(In1), Cluster15/1(In1), Cluster14/1(In1), Cluster13/1(In1), Cluster12/1(In1), Cluster11/1(In1), Cluster10/1(In1), Cluster9/1(In1), Cluster8/1(In1), Cluster7/1(In1), Cluster6/1(In1), Cluster5/1(In1), Cluster4/1(In1), Cluster3/1(In1), Cluster2/1(In1), Cluster1/1(In1)
  In1/1 -> Mux/1
  Mux/1 -> Interface/1(layerIn)

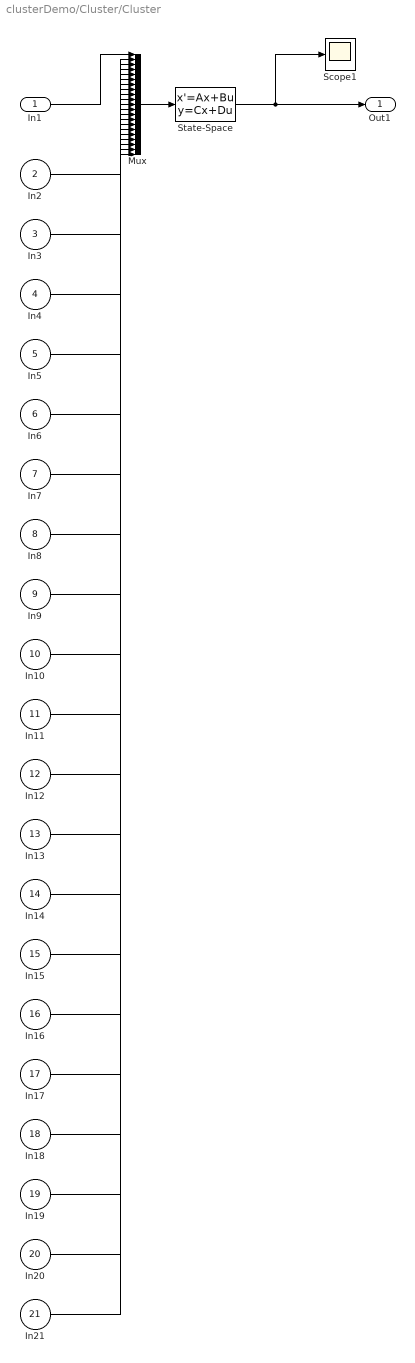
== system clusterDemo/Cluster/Cluster ==
  In1 : Inport  OutDataType=fixdt(1, 16)  OutScaling=2^0
  In2 : Inport  Port=2
  In3 : Inport  Port=3
  In4 : Inport  Port=4
  In5 : Inport  Port=5
  In6 : Inport  Port=6
  In7 : Inport  Port=7
  In8 : Inport  Port=8
  In9 : Inport  Port=9
  In10 : Inport  Port=10
  In11 : Inport  Port=11
  In12 : Inport  Port=12
  In13 : Inport  Port=13
  In14 : Inport  Port=14
  In15 : Inport  Port=15
  In16 : Inport  Port=16
  In17 : Inport  Port=17
  In18 : Inport  Port=18
  In19 : Inport  Port=19
  In20 : Inport  Port=20
  In21 : Inport  Port=21
  Mux : Mux  Inputs=21
  Scope1 : Scope
      settings: TimeRange=0.5847953216374258  YMin=-0.1657458563535892  YMax=1.21546961325967
  State-Space : StateSpace  A=A  B=B  C=C  D=D  X0=x0+var*rand(1)
  Out1 : Outport  OutDataType=fixdt(1, 16)  OutScaling=2^0
  wires:
  Mux/1 -> State-Space/1
  In1/1 -> Mux/1
  State-Space/1 -> Out1/1, Scope1/1
  In2/1 -> Mux/2
  In3/1 -> Mux/3
  In4/1 -> Mux/4
  In5/1 -> Mux/5
  In6/1 -> Mux/6
  In7/1 -> Mux/7
  In8/1 -> Mux/8
  In9/1 -> Mux/9
  In10/1 -> Mux/10
  In11/1 -> Mux/11
  In12/1 -> Mux/12
  In13/1 -> Mux/13
  In14/1 -> Mux/14
  In15/1 -> Mux/15
  In16/1 -> Mux/16
  In17/1 -> Mux/17
  In18/1 -> Mux/18
  In19/1 -> Mux/19
  In20/1 -> Mux/20
  In21/1 -> Mux/21

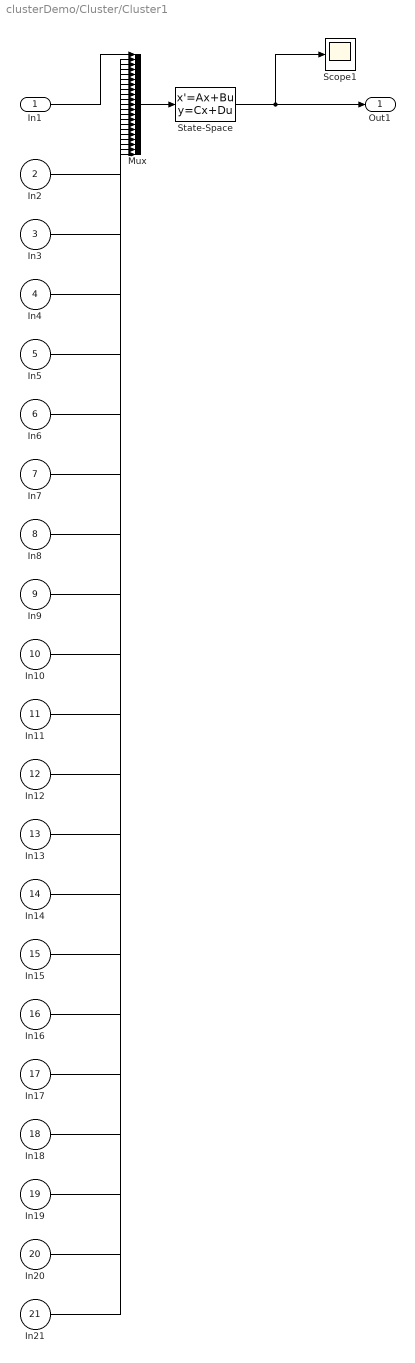
== system clusterDemo/Cluster/Cluster1 ==
  In1 : Inport  OutDataType=fixdt(1, 16)  OutScaling=2^0
  In2 : Inport  Port=2
  In3 : Inport  Port=3
  In4 : Inport  Port=4
  In5 : Inport  Port=5
  In6 : Inport  Port=6
  In7 : Inport  Port=7
  In8 : Inport  Port=8
  In9 : Inport  Port=9
  In10 : Inport  Port=10
  In11 : Inport  Port=11
  In12 : Inport  Port=12
  In13 : Inport  Port=13
  In14 : Inport  Port=14
  In15 : Inport  Port=15
  In16 : Inport  Port=16
  In17 : Inport  Port=17
  In18 : Inport  Port=18
  In19 : Inport  Port=19
  In20 : Inport  Port=20
  In21 : Inport  Port=21
  Mux : Mux  Inputs=21
  Scope1 : Scope
      settings: TimeRange=0.5847953216374258  YMin=-0.1657458563535892  YMax=1.21546961325967
  State-Space : StateSpace  A=A  B=B  C=C  D=D  X0=x0+var*rand(1)
  Out1 : Outport  OutDataType=fixdt(1, 16)  OutScaling=2^0
  wires:
  Mux/1 -> State-Space/1
  In1/1 -> Mux/1
  State-Space/1 -> Out1/1, Scope1/1
  In2/1 -> Mux/2
  In3/1 -> Mux/3
  In4/1 -> Mux/4
  In5/1 -> Mux/5
  In6/1 -> Mux/6
  In7/1 -> Mux/7
  In8/1 -> Mux/8
  In9/1 -> Mux/9
  In10/1 -> Mux/10
  In11/1 -> Mux/11
  In12/1 -> Mux/12
  In13/1 -> Mux/13
  In14/1 -> Mux/14
  In15/1 -> Mux/15
  In16/1 -> Mux/16
  In17/1 -> Mux/17
  In18/1 -> Mux/18
  In19/1 -> Mux/19
  In20/1 -> Mux/20
  In21/1 -> Mux/21

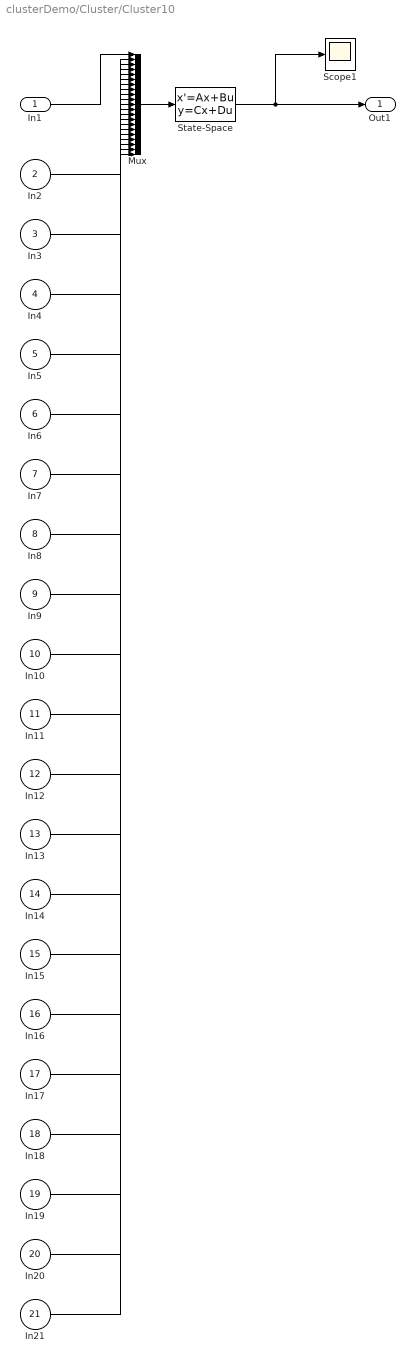
== system clusterDemo/Cluster/Cluster10 ==
  In1 : Inport  OutDataType=fixdt(1, 16)  OutScaling=2^0
  In2 : Inport  Port=2
  In3 : Inport  Port=3
  In4 : Inport  Port=4
  In5 : Inport  Port=5
  In6 : Inport  Port=6
  In7 : Inport  Port=7
  In8 : Inport  Port=8
  In9 : Inport  Port=9
  In10 : Inport  Port=10
  In11 : Inport  Port=11
  In12 : Inport  Port=12
  In13 : Inport  Port=13
  In14 : Inport  Port=14
  In15 : Inport  Port=15
  In16 : Inport  Port=16
  In17 : Inport  Port=17
  In18 : Inport  Port=18
  In19 : Inport  Port=19
  In20 : Inport  Port=20
  In21 : Inport  Port=21
  Mux : Mux  Inputs=21
  Scope1 : Scope
      settings: TimeRange=0.5847953216374258  YMin=-0.1657458563535892  YMax=1.21546961325967
  State-Space : StateSpace  A=A  B=B  C=C  D=D  X0=x0+var*rand(1)
  Out1 : Outport  OutDataType=fixdt(1, 16)  OutScaling=2^0
  wires:
  Mux/1 -> State-Space/1
  In1/1 -> Mux/1
  State-Space/1 -> Out1/1, Scope1/1
  In2/1 -> Mux/2
  In3/1 -> Mux/3
  In4/1 -> Mux/4
  In5/1 -> Mux/5
  In6/1 -> Mux/6
  In7/1 -> Mux/7
  In8/1 -> Mux/8
  In9/1 -> Mux/9
  In10/1 -> Mux/10
  In11/1 -> Mux/11
  In12/1 -> Mux/12
  In13/1 -> Mux/13
  In14/1 -> Mux/14
  In15/1 -> Mux/15
  In16/1 -> Mux/16
  In17/1 -> Mux/17
  In18/1 -> Mux/18
  In19/1 -> Mux/19
  In20/1 -> Mux/20
  In21/1 -> Mux/21

== system clusterDemo/Cluster/Cluster11 ==
  In1 : Inport  OutDataType=fixdt(1, 16)  OutScaling=2^0
  In2 : Inport  Port=2
  In3 : Inport  Port=3
  In4 : Inport  Port=4
  In5 : Inport  Port=5
  In6 : Inport  Port=6
  In7 : Inport  Port=7
  In8 : Inport  Port=8
  In9 : Inport  Port=9
  In10 : Inport  Port=10
  In11 : Inport  Port=11
  In12 : Inport  Port=12
  In13 : Inport  Port=13
  In14 : Inport  Port=14
  In15 : Inport  Port=15
  In16 : Inport  Port=16
  In17 : Inport  Port=17
  In18 : Inport  Port=18
  In19 : Inport  Port=19
  In20 : Inport  Port=20
  In21 : Inport  Port=21
  Mux : Mux  Inputs=21
  Scope1 : Scope
      settings: TimeRange=0.5847953216374258  YMin=-0.1657458563535892  YMax=1.21546961325967
  State-Space : StateSpace  A=A  B=B  C=C  D=D  X0=x0+var*rand(1)
  Out1 : Outport  OutDataType=fixdt(1, 16)  OutScaling=2^0
  wires:
  Mux/1 -> State-Space/1
  In1/1 -> Mux/1
  State-Space/1 -> Out1/1, Scope1/1
  In2/1 -> Mux/2
  In3/1 -> Mux/3
  In4/1 -> Mux/4
  In5/1 -> Mux/5
  In6/1 -> Mux/6
  In7/1 -> Mux/7
  In8/1 -> Mux/8
  In9/1 -> Mux/9
  In10/1 -> Mux/10
  In11/1 -> Mux/11
  In12/1 -> Mux/12
  In13/1 -> Mux/13
  In14/1 -> Mux/14
  In15/1 -> Mux/15
  In16/1 -> Mux/16
  In17/1 -> Mux/17
  In18/1 -> Mux/18
  In19/1 -> Mux/19
  In20/1 -> Mux/20
  In21/1 -> Mux/21

== system clusterDemo/Cluster/Cluster12 ==
  In1 : Inport  OutDataType=fixdt(1, 16)  OutScaling=2^0
  In2 : Inport  Port=2
  In3 : Inport  Port=3
  In4 : Inport  Port=4
  In5 : Inport  Port=5
  In6 : Inport  Port=6
  In7 : Inport  Port=7
  In8 : Inport  Port=8
  In9 : Inport  Port=9
  In10 : Inport  Port=10
  In11 : Inport  Port=11
  In12 : Inport  Port=12
  In13 : Inport  Port=13
  In14 : Inport  Port=14
  In15 : Inport  Port=15
  In16 : Inport  Port=16
  In17 : Inport  Port=17
  In18 : Inport  Port=18
  In19 : Inport  Port=19
  In20 : Inport  Port=20
  In21 : Inport  Port=21
  Mux : Mux  Inputs=21
  Scope1 : Scope
      settings: TimeRange=0.5847953216374258  YMin=-0.1657458563535892  YMax=1.21546961325967
  State-Space : StateSpace  A=A  B=B  C=C  D=D  X0=x0+var*rand(1)
  Out1 : Outport  OutDataType=fixdt(1, 16)  OutScaling=2^0
  wires:
  Mux/1 -> State-Space/1
  In1/1 -> Mux/1
  State-Space/1 -> Out1/1, Scope1/1
  In2/1 -> Mux/2
  In3/1 -> Mux/3
  In4/1 -> Mux/4
  In5/1 -> Mux/5
  In6/1 -> Mux/6
  In7/1 -> Mux/7
  In8/1 -> Mux/8
  In9/1 -> Mux/9
  In10/1 -> Mux/10
  In11/1 -> Mux/11
  In12/1 -> Mux/12
  In13/1 -> Mux/13
  In14/1 -> Mux/14
  In15/1 -> Mux/15
  In16/1 -> Mux/16
  In17/1 -> Mux/17
  In18/1 -> Mux/18
  In19/1 -> Mux/19
  In20/1 -> Mux/20
  In21/1 -> Mux/21

== system clusterDemo/Cluster/Cluster13 ==
  In1 : Inport  OutDataType=fixdt(1, 16)  OutScaling=2^0
  In2 : Inport  Port=2
  In3 : Inport  Port=3
  In4 : Inport  Port=4
  In5 : Inport  Port=5
  In6 : Inport  Port=6
  In7 : Inport  Port=7
  In8 : Inport  Port=8
  In9 : Inport  Port=9
  In10 : Inport  Port=10
  In11 : Inport  Port=11
  In12 : Inport  Port=12
  In13 : Inport  Port=13
  In14 : Inport  Port=14
  In15 : Inport  Port=15
  In16 : Inport  Port=16
  In17 : Inport  Port=17
  In18 : Inport  Port=18
  In19 : Inport  Port=19
  In20 : Inport  Port=20
  In21 : Inport  Port=21
  Mux : Mux  Inputs=21
  Scope1 : Scope
      settings: TimeRange=0.5847953216374258  YMin=-0.1657458563535892  YMax=1.21546961325967
  State-Space : StateSpace  A=A  B=B  C=C  D=D  X0=x0+var*rand(1)
  Out1 : Outport  OutDataType=fixdt(1, 16)  OutScaling=2^0
  wires:
  Mux/1 -> State-Space/1
  In1/1 -> Mux/1
  State-Space/1 -> Out1/1, Scope1/1
  In2/1 -> Mux/2
  In3/1 -> Mux/3
  In4/1 -> Mux/4
  In5/1 -> Mux/5
  In6/1 -> Mux/6
  In7/1 -> Mux/7
  In8/1 -> Mux/8
  In9/1 -> Mux/9
  In10/1 -> Mux/10
  In11/1 -> Mux/11
  In12/1 -> Mux/12
  In13/1 -> Mux/13
  In14/1 -> Mux/14
  In15/1 -> Mux/15
  In16/1 -> Mux/16
  In17/1 -> Mux/17
  In18/1 -> Mux/18
  In19/1 -> Mux/19
  In20/1 -> Mux/20
  In21/1 -> Mux/21

== system clusterDemo/Cluster/Cluster14 ==
  In1 : Inport  OutDataType=fixdt(1, 16)  OutScaling=2^0
  In2 : Inport  Port=2
  In3 : Inport  Port=3
  In4 : Inport  Port=4
  In5 : Inport  Port=5
  In6 : Inport  Port=6
  In7 : Inport  Port=7
  In8 : Inport  Port=8
  In9 : Inport  Port=9
  In10 : Inport  Port=10
  In11 : Inport  Port=11
  In12 : Inport  Port=12
  In13 : Inport  Port=13
  In14 : Inport  Port=14
  In15 : Inport  Port=15
  In16 : Inport  Port=16
  In17 : Inport  Port=17
  In18 : Inport  Port=18
  In19 : Inport  Port=19
  In20 : Inport  Port=20
  In21 : Inport  Port=21
  Mux : Mux  Inputs=21
  Scope1 : Scope
      settings: TimeRange=0.5847953216374258  YMin=-0.1657458563535892  YMax=1.21546961325967
  State-Space : StateSpace  A=A  B=B  C=C  D=D  X0=x0+var*rand(1)
  Out1 : Outport  OutDataType=fixdt(1, 16)  OutScaling=2^0
  wires:
  Mux/1 -> State-Space/1
  In1/1 -> Mux/1
  State-Space/1 -> Out1/1, Scope1/1
  In2/1 -> Mux/2
  In3/1 -> Mux/3
  In4/1 -> Mux/4
  In5/1 -> Mux/5
  In6/1 -> Mux/6
  In7/1 -> Mux/7
  In8/1 -> Mux/8
  In9/1 -> Mux/9
  In10/1 -> Mux/10
  In11/1 -> Mux/11
  In12/1 -> Mux/12
  In13/1 -> Mux/13
  In14/1 -> Mux/14
  In15/1 -> Mux/15
  In16/1 -> Mux/16
  In17/1 -> Mux/17
  In18/1 -> Mux/18
  In19/1 -> Mux/19
  In20/1 -> Mux/20
  In21/1 -> Mux/21

== system clusterDemo/Cluster/Cluster15 ==
  In1 : Inport  OutDataType=fixdt(1, 16)  OutScaling=2^0
  In2 : Inport  Port=2
  In3 : Inport  Port=3
  In4 : Inport  Port=4
  In5 : Inport  Port=5
  In6 : Inport  Port=6
  In7 : Inport  Port=7
  In8 : Inport  Port=8
  In9 : Inport  Port=9
  In10 : Inport  Port=10
  In11 : Inport  Port=11
  In12 : Inport  Port=12
  In13 : Inport  Port=13
  In14 : Inport  Port=14
  In15 : Inport  Port=15
  In16 : Inport  Port=16
  In17 : Inport  Port=17
  In18 : Inport  Port=18
  In19 : Inport  Port=19
  In20 : Inport  Port=20
  In21 : Inport  Port=21
  Mux : Mux  Inputs=21
  Scope1 : Scope
      settings: TimeRange=0.5847953216374258  YMin=-0.1657458563535892  YMax=1.21546961325967
  State-Space : StateSpace  A=A  B=B  C=C  D=D  X0=x0+var*rand(1)
  Out1 : Outport  OutDataType=fixdt(1, 16)  OutScaling=2^0
  wires:
  Mux/1 -> State-Space/1
  In1/1 -> Mux/1
  State-Space/1 -> Out1/1, Scope1/1
  In2/1 -> Mux/2
  In3/1 -> Mux/3
  In4/1 -> Mux/4
  In5/1 -> Mux/5
  In6/1 -> Mux/6
  In7/1 -> Mux/7
  In8/1 -> Mux/8
  In9/1 -> Mux/9
  In10/1 -> Mux/10
  In11/1 -> Mux/11
  In12/1 -> Mux/12
  In13/1 -> Mux/13
  In14/1 -> Mux/14
  In15/1 -> Mux/15
  In16/1 -> Mux/16
  In17/1 -> Mux/17
  In18/1 -> Mux/18
  In19/1 -> Mux/19
  In20/1 -> Mux/20
  In21/1 -> Mux/21

== system clusterDemo/Cluster/Cluster16 ==
  In1 : Inport  OutDataType=fixdt(1, 16)  OutScaling=2^0
  In2 : Inport  Port=2
  In3 : Inport  Port=3
  In4 : Inport  Port=4
  In5 : Inport  Port=5
  In6 : Inport  Port=6
  In7 : Inport  Port=7
  In8 : Inport  Port=8
  In9 : Inport  Port=9
  In10 : Inport  Port=10
  In11 : Inport  Port=11
  In12 : Inport  Port=12
  In13 : Inport  Port=13
  In14 : Inport  Port=14
  In15 : Inport  Port=15
  In16 : Inport  Port=16
  In17 : Inport  Port=17
  In18 : Inport  Port=18
  In19 : Inport  Port=19
  In20 : Inport  Port=20
  In21 : Inport  Port=21
  Mux : Mux  Inputs=21
  Scope1 : Scope
      settings: TimeRange=0.5847953216374258  YMin=-0.1657458563535892  YMax=1.21546961325967
  State-Space : StateSpace  A=A  B=B  C=C  D=D  X0=x0+var*rand(1)
  Out1 : Outport  OutDataType=fixdt(1, 16)  OutScaling=2^0
  wires:
  Mux/1 -> State-Space/1
  In1/1 -> Mux/1
  State-Space/1 -> Out1/1, Scope1/1
  In2/1 -> Mux/2
  In3/1 -> Mux/3
  In4/1 -> Mux/4
  In5/1 -> Mux/5
  In6/1 -> Mux/6
  In7/1 -> Mux/7
  In8/1 -> Mux/8
  In9/1 -> Mux/9
  In10/1 -> Mux/10
  In11/1 -> Mux/11
  In12/1 -> Mux/12
  In13/1 -> Mux/13
  In14/1 -> Mux/14
  In15/1 -> Mux/15
  In16/1 -> Mux/16
  In17/1 -> Mux/17
  In18/1 -> Mux/18
  In19/1 -> Mux/19
  In20/1 -> Mux/20
  In21/1 -> Mux/21
